simulink model "DiscModeController"  (Simulink 7.7)
settings: Solver=ode45  StartTime=0.0  StopTime=10.0  RelTol=1e-3
settings Model: Creator=jporter  LastModifiedBy=jporter

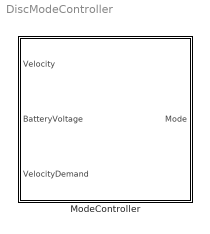
== system DiscModeController ==
  ModeController : Subsystem

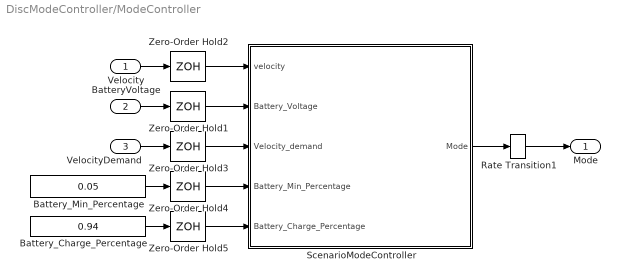
== system DiscModeController/ModeController ==
  Velocity : Inport
  BatteryVoltage : Inport  Port=2
  VelocityDemand : Inport  Port=3
  " Battery_Charge_Percentage" : Constant  Value=0.94
  Battery_Min_Percentage : Constant  Value=0.05
  Rate Transition1 : RateTransition  OutPortSampleTime=0
  ScenarioModeController : Stateflow chart  TreatAsAtomicUnit=on
  Zero-Order Hold{1..5} (5 alike) : ZeroOrderHold  Priority=-1  SampleTime=0.1
  Mode : Outport
  wires:
  Velocity/1 -> Zero-Order Hold2/1
  BatteryVoltage/1 -> Zero-Order Hold1/1
  VelocityDemand/1 -> Zero-Order Hold3/1
  ScenarioModeController/1(Mode) -> Rate Transition1/1
  Battery_Min_Percentage/1 -> Zero-Order Hold4/1
  " Battery_Charge_Percentage"/1 -> Zero-Order Hold5/1
  Zero-Order Hold2/1 -> ScenarioModeController/1(velocity)
  Zero-Order Hold1/1 -> ScenarioModeController/2(Battery_Voltage)
  Zero-Order Hold3/1 -> ScenarioModeController/3(Velocity_demand)
  Zero-Order Hold4/1 -> ScenarioModeController/4(Battery_Min_Percentage)
  Zero-Order Hold5/1 -> ScenarioModeController/5(Battery_Charge_Percentage)
  Rate Transition1/1 -> Mode/1

== matlab function ModeController/ScenarioModeController ==
  data: velocity input double; Mode output double; Battery_Voltage input double; Velocity_demand input double; Battery_Min_Percentage input double; Battery_Charge_Percentage input double
function Mode  = fcn(velocity, Battery_Voltage, Velocity_demand, Battery_Min_Percentage, Battery_Charge_Percentage)
%#eml
if Battery_Voltage < 200*Battery_Min_Percentage
    Mode = 1; % DE ON, Battery charge
elseif velocity < Velocity_demand
    Mode = 0; % we need all energy   
elseif Battery_Voltage < 200*Battery_Charge_Percentage
    Mode = 1; % charge
else
    Mode = 2; % DE ON, Battery is disconnected
end

%Mode = 2; % DE ON, Battery is disconnected
